simulink model "throttle_model"  (R2025b)
settings: Solver=VariableStepAuto  StartTime=0.0  StopTime=8.0  RelTol=1e-3
libraries: slpidlib x1
settings Model: Creator=91931  LastModifiedBy=91931

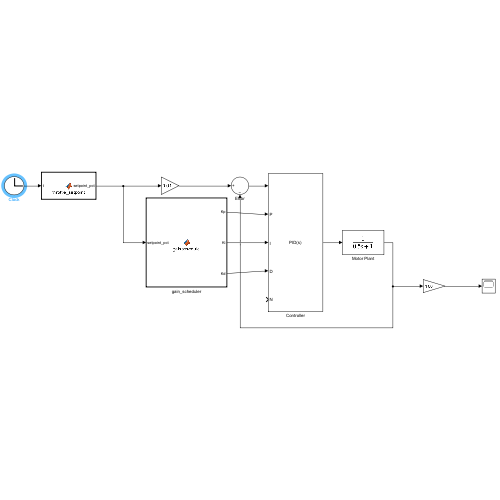
[thumbnail: Simulink's stored preview of the top-level diagram]
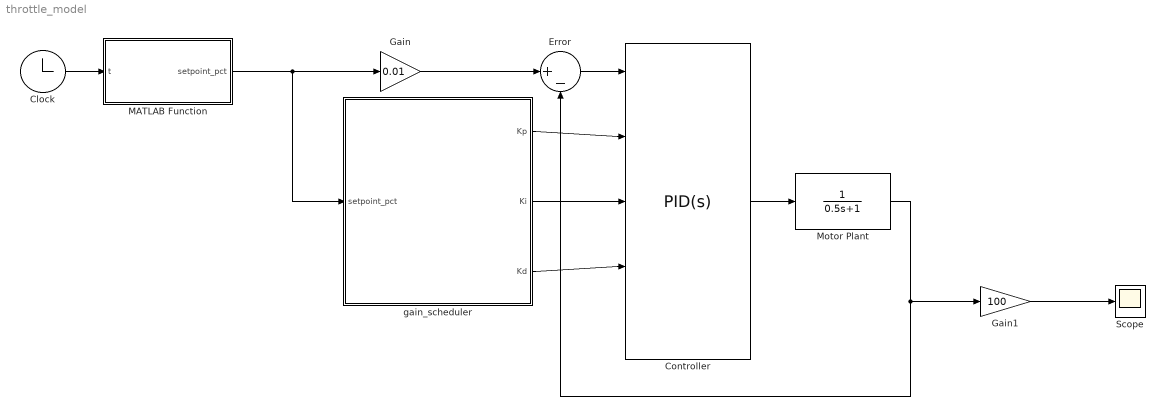
== system throttle_model ==
  Clock : Clock
  Controller : slpidlib/PID Controller  Controller=PID  Form=Parallel  TimeDomain=Continuous-time  UseExternalTs=off  SampleTime=-1  IntegratorMethod=Forward Euler  FilterMethod=Forward Euler  ControllerParametersSource=external  P=1  I=1  UseKiTs=off  D=0  UseExternalDerivativeSource=off  N=100  UseFilter=on  TunerSelectOption=Transfer Function Based (PID Tuner App)  InitialConditionSource=internal  InitialConditionForIntegrator=0  InitialConditionForFilter=0  DifferentiatorICPrevScaledInput=0  ExternalReset=none  TrackingMode=off  Kt=1  LimitOutput=off  SatLimitsSource=internal  UpperSaturationLimit=inf  LowerSaturationLimit=-inf  LinearizeAsGain=on  AntiWindupMode=none  Kb=1  LimitIntegrator=off  UpperIntegratorSaturationLimit=inf  LowerIntegratorSaturationLimit=-inf  POutMin=[]  POutMax=[]  IOutMin=[]  IOutMax=[]  DOutMin=[]  DOutMax=[]  NOutMin=[]  NOutMax=[]  SumOutMin=[]  SumOutMax=[]  SaturationOutMin=[]  SaturationOutMax=[]  PParamMin=[]  PParamMax=[]  IParamMin=[]  IParamMax=[]  DParamMin=[]  DParamMax=[]  NParamMin=[]  NParamMax=[]  KbParamMin=[]  KbParamMax=[]  KtParamMin=[]  KtParamMax=[]  KbOutMin=[]  KbOutMax=[]  KtOutMin=[]  KtOutMax=[]  IntegratorOutMin=[]  IntegratorOutMax=[]  FilterOutMin=[]  FilterOutMax=[]  SumI1OutMin=[]  SumI1OutMax=[]  SumI2OutMin=[]  SumI2OutMax=[]  SumI3OutMin=[]  SumI3OutMax=[]  SumI4OutMin=[]  SumI4OutMax=[]  SumDOutMin=[]  SumDOutMax=[]  DifferentiatorOutMin=[]  DifferentiatorOutMax=[]  FilterDiffOutCoefMin=[]  FilterDiffOutCoefMax=[]  ReciprocalOutMin=[]  ReciprocalOutMax=[]  SumDenOutMin=[]  SumDenOutMax=[]  SumNumOutMin=[]  SumNumOutMax=[]  DivideOutMin=[]  DivideOutMax=[]  UdiffTsProdOutMin=[]  UdiffTsProdOutMax=[]  NTsProdOutMin=[]  NTsProdOutMax=[]  UintegralTsProdOutMin=[]  UintegralTsProdOutMax=[]  UngainTsProdOutMin=[]  UngainTsProdOutMax=[]  ClampingZeroOutDataTypeStr=Inherit: Inherit via back propagation  ClampingZeroOutMin=[]  ClampingZeroOutMax=[]  FilterDenConstantOutDataTypeStr=Inherit: Inherit via back propagation  FilterDenConstantOutMin=[]  FilterDenConstantOutMax=[]  PCopyOutDataTypeStr=Inherit: Inherit via back propagation  PCopyOutMin=[]  PCopyOutMax=[]  NCopyOutDataTypeStr=Inherit: Inherit via back propagation  NCopyOutMin=[]  NCopyOutMax=[]  IntegratorContinuousStateAttributes=''  IntegratorStateMustResolveToSignalObject=off  IntegratorRTWStateStorageClass=Auto  FilterContinuousStateAttributes=''  FilterStateMustResolveToSignalObject=off  FilterRTWStateStorageClass=Auto  ParallelPVariant=ExternalParameters  IdealPVariant=Disabled  IVariant=ExternalParameters  DVariant=ExternalParameters  IntegratorVariant=Continuous  SatVariant=Disabled  AWVariant=Passthrough  PCopyVariant=Disabled  TRVariant=Disabled  FdbkBlocksVariant=Forward  IdealPFdbkVariant=Disabled  SatFdbkVariant=Disabled  DerivativeFilterVariant=ContFilter  NVariant=ExternalParameters  NCopyVariant=Disabled  FilterICVariant=InternalICsFilter  IntegratorICVariant=InternalICs  ExternalResetVariant=Disabled  TRSumVariant=Passthrough  SumFdbkVariant=Disabled  SumVariant=Sum_PID  TsampFilterVariant=InternalTs  TsampNgainVariant=Passthrough  TsampIntegralVariant=Disabled_SignalSpec  ExternalSaturationOutDataTypeStr=Inherit: Same as second input  DerivativeSourceVariant=ErrorSignal  PreIntVariant=InternalPreInt
  Error : Sum  Inputs=|+-
  Gain : Gain  Gain=0.01
  Gain1 : Gain  Gain=100
  MATLAB Function : MATLAB Function  TreatAsAtomicUnit=on
  Motor Plant : TransferFcn  Denominator=[0.5 1]
  Scope : Scope
      settings: ActiveDisplayYMinimum=-2.0406352783616626  ActiveDisplayYMaximum=123.60622792997265
  gain_scheduler : MATLAB Function  TreatAsAtomicUnit=on
  wires:
  MATLAB Function/1(setpoint_pct) -> gain_scheduler/1(setpoint_pct), Gain/1
  Gain/1 -> Error/1
  gain_scheduler/1(Kp) -> Controller/2
  gain_scheduler/2(Ki) -> Controller/3
  gain_scheduler/3(Kd) -> Controller/4
  Error/1 -> Controller/1
  Controller/1 -> Motor Plant/1
  Motor Plant/1 -> Error/2, Gain1/1
  Gain1/1 -> Scope/1
  Clock/1 -> MATLAB Function/1(t)

== matlab function throttle_model/gain_scheduler ==
  data: setpoint_pct input; Kp output; Ki output; Kd output
function [Kp, Ki, Kd] = gainschedule(setpoint_pct)
% Gains for three throttle zones (0-30%, 30-70%, 70-100%)
persistent zone_gains thresholds
if isempty(zone_gains)
    thresholds = [30, 70];          % zone boundaries
    % Gains: [Kp, Ki, Kd] for each zone
    zone_gains = [0.58, 2.58, 0.00;   % Zone 1: low
                  2.13, 8.26, 0.00;  % Zone 2: mid
                  4.70, 19.79, 0.00];  % Zone 3: high
end

if setpoint_pct <= thresholds(1)
    zone = 1;
elseif setpoint_pct <= thresholds(2)
    zone = 2;
else
    zone = 3;
end

Kp = zone_gains(zone, 1);
Ki = zone_gains(zone, 2);
Kd = zone_gains(zone, 3);
end

== matlab function throttle_model/MATLAB Function ==
  data: t input; setpoint_pct output
function setpoint_pct = throttle_setpoint(t)
% Generate throttle setpoint (percent) based on simulation time
% Time intervals:
%   0 <= t < 2  → 20%
%   2 <= t < 4  → 50%
%   t >= 4      → 85%
if t < 2
    setpoint_pct = 20;
elseif t < 4
    setpoint_pct = 50;
else
    setpoint_pct = 85;
end
end
